simulink model "NONLINEAR_CASE_simulation"  (R2022b)
settings: Solver=ode3  StartTime=0.0  StopTime=15  FixedStep=1e-4  RelTol=1e-6  EnableMultiTasking=on
settings Model: Creator=sf  LastModifiedBy=sf
settings ModelReferenceCC: EnableRefExpFcnMdlSchedulingChecks=on

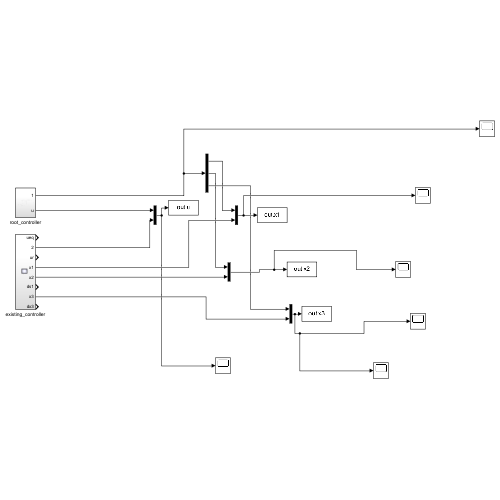
[thumbnail: Simulink's stored preview of the top-level diagram]
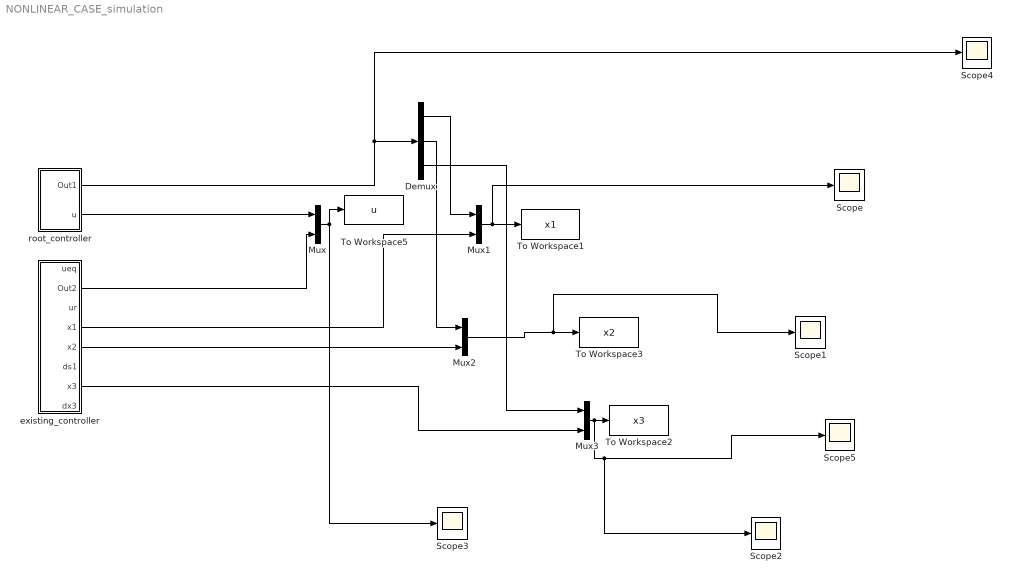
== system NONLINEAR_CASE_simulation ==
  Demux : Demux  Outputs=3
  Mux{,1..3} (4 alike) : Mux  Inputs=2
  Scope{,1..5} (6 alike) : Scope
  To Workspace1 : ToWorkspace  VariableName=x1  SampleTime=-1
  To Workspace2 : ToWorkspace  VariableName=x3  SampleTime=-1
  To Workspace3 : ToWorkspace  VariableName=x2  SampleTime=-1
  To Workspace5 : ToWorkspace  VariableName=u  SampleTime=-1
  existing_controller : Subsystem
  root_controller : Subsystem
  wires:
  root_controller/1(Out1) -> Scope4/1, Demux/1
  root_controller/2(u) -> Mux/1
  existing_controller/2(Out2) -> Mux/2
  existing_controller/4(x1) -> Mux1/2
  Mux/1 -> Scope3/1, To Workspace5/1
  Demux/1 -> Mux1/1
  Demux/2 -> Mux2/1
  existing_controller/5(x2) -> Mux2/2
  Mux2/1 -> Scope1/1, To Workspace3/1
  Demux/3 -> Mux3/1
  existing_controller/7(x3) -> Mux3/2
  Mux3/1 -> Scope2/1, Scope5/1, To Workspace2/1
  Mux1/1 -> Scope/1, To Workspace1/1

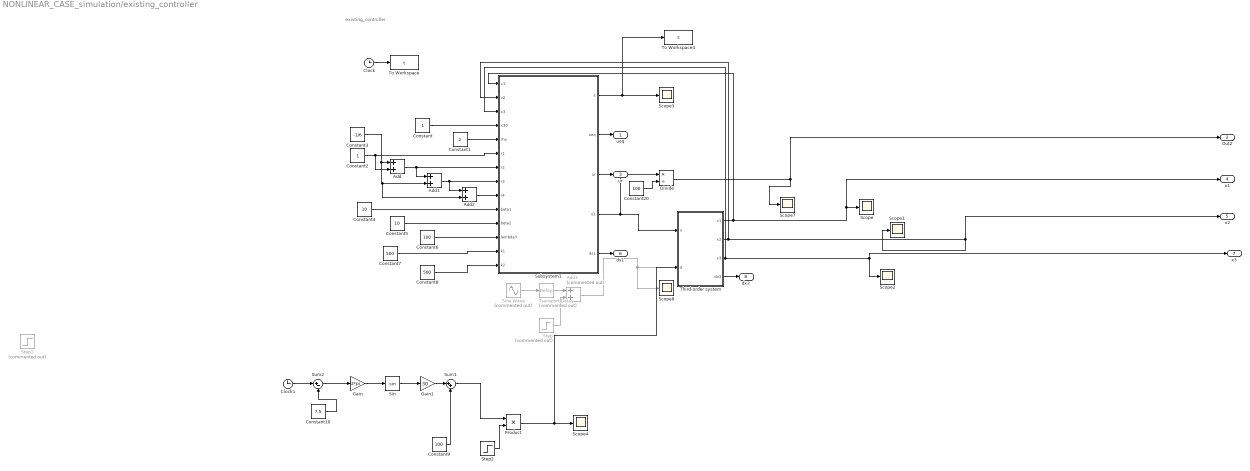
== system NONLINEAR_CASE_simulation/existing_controller ==
  note: existing_controller
  Add : Sum
  Add1 : Sum
  Add2 : Sum
  Add3 : Sum  Commented=on
  Clock : Clock
  Clock1 : Clock
  Constant : Constant
  Constant1 : Constant  Value=2
  Constant10 : Constant  Value=7.5
  Constant2 : Constant
  Constant20 : Constant  Value=100
  Constant3 : Constant  Value=-1/6
  Constant4 : Constant  Value=10
  Constant5 : Constant  Value=10
  Constant6 : Constant  Value=100
  Constant7 : Constant  Value=500
  Constant8 : Constant  Value=500
  Constant9 : Constant  Value=100
  Divide : Product  Inputs=*/
  Gain : Gain  Gain=2*pi
  Gain1 : Gain  Gain=30
  Product : Product
  Scope{,1..4,7..8} (7 alike) : Scope
  Sin : Trigonometry
  Sine Wave : Sin  Commented=on  Amplitude=30  Bias=100  Frequency=2*pi  SampleTime=0
  Step : Step  Commented=on  Time=7.5  After=0  SampleTime=0
  Step1 : Step  Commented=on  Time=7.5  After=0  SampleTime=0
  Step2 : Step  Time=7.5  SampleTime=0
  Subsystem1 : Subsystem
  Sum1 : Sum  Inputs=|++
  Sum2 : Sum  Inputs=|+-
  Third-order system : Subsystem
  To Workspace : ToWorkspace  VariableName=t  SampleTime=-1
  To Workspace4 : ToWorkspace  VariableName=s  SampleTime=-1
  Transport Delay : TransportDelay  Commented=on  DelayTime=7.5
  ueq : Outport
  Out2 : Outport  Port=2
  ur : Outport  Port=3
  x1 : Outport  Port=4
  x2 : Outport  Port=5
  ds1 : Outport  Port=6
  x3 : Outport  Port=7
  dx3 : Outport  Port=8
  wires:
  Third-order system/3(x3) -> x3/1, Scope2/1, Subsystem1/3(x3)
  Subsystem1/3(ur) -> ur/1
  Add/1 -> Add1/1, Subsystem1/7(r2)
  Constant3/1 -> Add2/2, Add1/2, Add/1
  Constant/1 -> Subsystem1/4(x30)
  Constant8/1 -> Subsystem1/14(k2)
  Third-order system/4(dx3) -> dx3/1
  Constant2/1 -> Subsystem1/6(r1), Add/2
  Third-order system/2(x2) -> x2/1, Scope1/1, Subsystem1/2(x2)
  Constant5/1 -> Subsystem1/11(beta2)
  Constant7/1 -> Subsystem1/13(k1)
  Third-order system/1(x1) -> x1/1, Scope/1, Subsystem1/1(x1)
  Subsystem1/4(u1) -> Divide/1, Third-order system/1(u)
  Step/1 -> Add3/2
  Add2/1 -> Subsystem1/9(r4)
  Divide/1 -> Out2/1, Scope7/1
  Constant20/1 -> Divide/2
  Add3/1 -> Scope8/1
  Sine Wave/1 -> Transport Delay/1
  Add1/1 -> Add2/1, Subsystem1/8(r3)
  Constant6/1 -> Subsystem1/12(lambda3)
  Constant1/1 -> Subsystem1/5(rho)
  Subsystem1/1(s) -> To Workspace4/1, Scope3/1
  Transport Delay/1 -> Add3/1
  Clock/1 -> To Workspace/1
  Constant4/1 -> Subsystem1/10(beta1)
  Subsystem1/2(ueq) -> ueq/1
  Subsystem1/5(ds1) -> ds1/1
  Gain/1 -> Sin/1
  Sum1/1 -> Product/1
  Product/1 -> Third-order system/2(d), Scope4/1
  Gain1/1 -> Sum1/1
  Sum2/1 -> Gain/1
  Step2/1 -> Product/2
  Constant9/1 -> Sum1/2
  Sin/1 -> Gain1/1
  Constant10/1 -> Sum2/2
  Clock1/1 -> Sum2/1

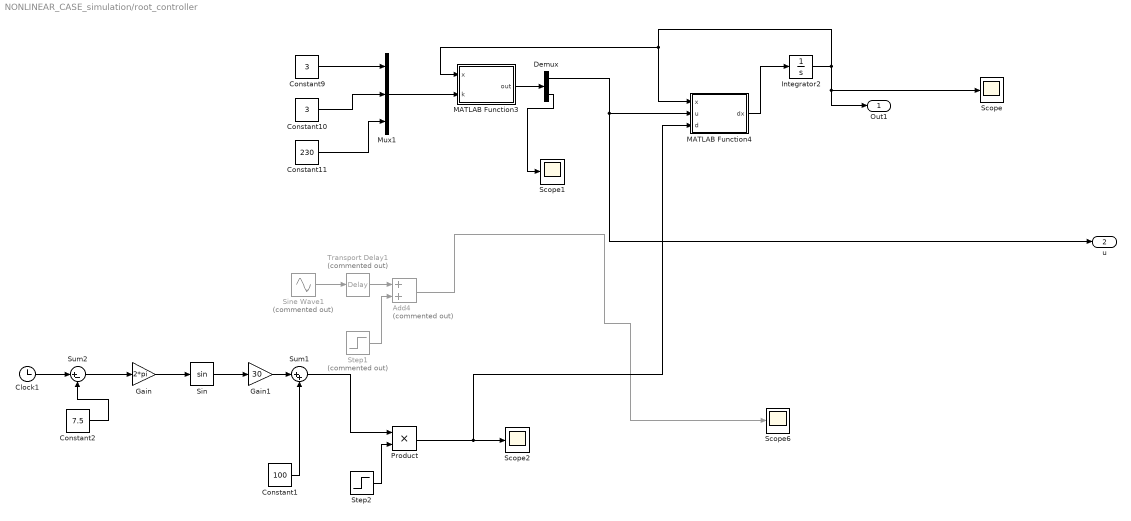
== system NONLINEAR_CASE_simulation/root_controller ==
  Add4 : Sum  Commented=on
  Clock1 : Clock
  Constant1 : Constant  Value=100
  Constant10 : Constant  Value=3
  Constant11 : Constant  Value=230
  Constant2 : Constant  Value=7.5
  Constant9 : Constant  Value=3
  Demux : Demux  Outputs=[1 7]
  Gain : Gain  Gain=2*pi
  Gain1 : Gain  Gain=30
  Integrator2 : Integrator  InitialCondition=[1;1;1]
  MATLAB Function3 : MATLAB Function  TreatAsAtomicUnit=on
  MATLAB Function4 : MATLAB Function  TreatAsAtomicUnit=on
  Mux1 : Mux  Inputs=3
  Product : Product
  Scope{,1..2,6} (4 alike) : Scope
  Sin : Trigonometry
  Sine Wave1 : Sin  Commented=on  Amplitude=30  Bias=100  Frequency=2*pi  SampleTime=0
  Step1 : Step  Commented=on  Time=7.5  After=0  SampleTime=0
  Step2 : Step  Time=7.5  SampleTime=0
  Sum1 : Sum  Inputs=|++
  Sum2 : Sum  Inputs=|+-
  Transport Delay1 : TransportDelay  Commented=on  DelayTime=7.5
  Out1 : Outport
  u : Outport  Port=2
  wires:
  Integrator2/1 -> Scope/1, Out1/1, MATLAB Function3/1(x), MATLAB Function4/1(x)
  Constant11/1 -> Mux1/3
  Constant10/1 -> Mux1/2
  Add4/1 -> Scope6/1
  Constant9/1 -> Mux1/1
  Demux/1 -> u/1, MATLAB Function4/2(u)
  Mux1/1 -> MATLAB Function3/2(k)
  MATLAB Function4/1(dx) -> Integrator2/1
  Sine Wave1/1 -> Transport Delay1/1
  Transport Delay1/1 -> Add4/1
  Step1/1 -> Add4/2
  MATLAB Function3/1(out) -> Demux/1
  Demux/2 -> Scope1/1
  Sin/1 -> Gain1/1
  Constant1/1 -> Sum1/2
  Gain1/1 -> Sum1/1
  Product/1 -> MATLAB Function4/3(d), Scope2/1
  Clock1/1 -> Sum2/1
  Step2/1 -> Product/2
  Constant2/1 -> Sum2/2
  Sum2/1 -> Gain/1
  Sum1/1 -> Product/1
  Gain/1 -> Sin/1

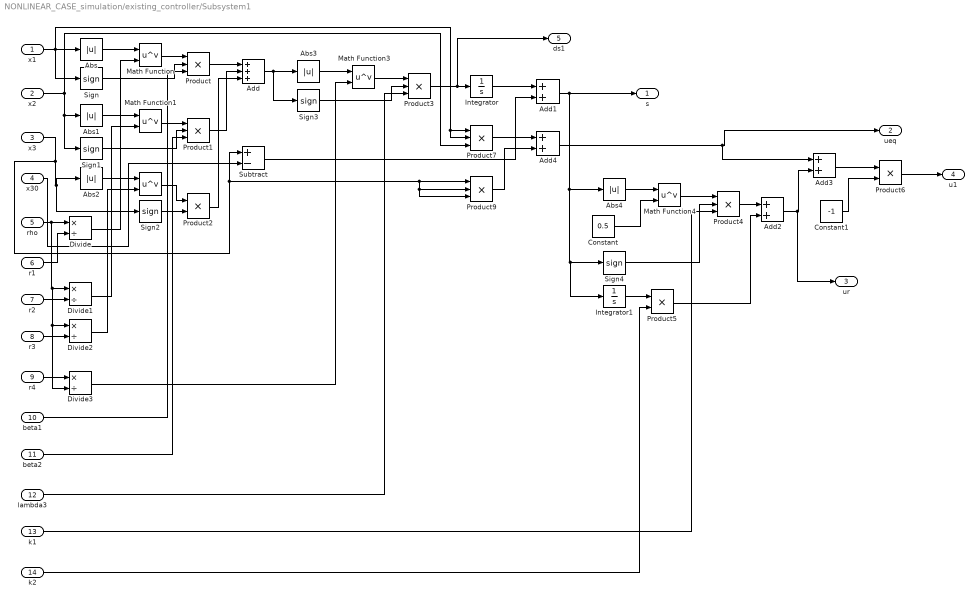
== system NONLINEAR_CASE_simulation/existing_controller/Subsystem1 ==
  x1 : Inport
  x2 : Inport  Port=2
  x3 : Inport  Port=3
  x30 : Inport  Port=4
  rho : Inport  Port=5
  r1 : Inport  Port=6
  r2 : Inport  Port=7
  r3 : Inport  Port=8
  r4 : Inport  Port=9
  beta1 : Inport  Port=10
  beta2 : Inport  Port=11
  lambda3 : Inport  Port=12
  k1 : Inport  Port=13
  k2 : Inport  Port=14
  " " : Math  Operator=pow  SignedPower=on
  Abs{,1..4} (5 alike) : Abs  SaturateOnIntegerOverflow=off
  Add : Sum  Inputs=+++
  Add{1..4} (4 alike) : Sum
  Constant : Constant  Value=0.5
  Constant1 : Constant  Value=-1
  Divide{,1..3} (4 alike) : Product  Inputs=*/
  Integrator : Integrator
  Integrator1 : Integrator
  Math Function{,1,3..4} (4 alike) : Math  Operator=pow  SignedPower=on
  Product{,1,3..4,7,9} (6 alike) : Product  Inputs=3
  Product2 : Product
  Product5 : Product
  Product6 : Product
  Sign{,1..4} (5 alike) : Signum
  Subtract : Sum  Inputs=+-
  s : Outport
  ueq : Outport  Port=2
  ur : Outport  Port=3
  u1 : Outport  Port=4
  ds1 : Outport  Port=5
  wires:
  k2/1 -> Product5/2
  Add3/1 -> Product6/1
  Constant/1 -> Math Function4/2
  x1/1 -> Sign/1, Product7/2, Product7/1, Abs/1
  lambda3/1 -> Product3/3
  Math Function4/1 -> Product4/1
  Constant1/1 -> Product6/2
  Abs4/1 -> Math Function4/1
  Abs/1 -> Math Function/1
  Math Function/1 -> Product/1
  Sign1/1 -> Product1/2
  Divide3/1 -> Math Function3/2
  " "/1 -> Product2/1
  rho/1 -> Divide3/2, Divide2/1, Divide1/1, Divide/1
  Abs3/1 -> Math Function3/1
  Abs2/1 -> " "/1
  Sign2/1 -> Product2/2
  Product1/1 -> Add/2
  r1/1 -> Divide/2
  r3/1 -> Divide2/2
  x2/1 -> Sign1/1, Abs1/1, Product7/3
  beta2/1 -> Product1/3
  x3/1 -> Product9/3, Product9/2, Product9/1, Subtract/1, Sign2/1, Abs2/1
  Abs1/1 -> Math Function1/1
  Product/1 -> Add/1
  Divide2/1 -> " "/2
  Add/1 -> Sign3/1, Abs3/1
  Product2/1 -> Add/3
  Sign4/1 -> Product4/2
  Product5/1 -> Add2/2
  Sign3/1 -> Product3/2
  Product4/1 -> Add2/1
  Integrator/1 -> Add1/1
  r4/1 -> Divide3/1
  Integrator1/1 -> Product5/1
  Math Function3/1 -> Product3/1
  Product3/1 -> ds1/1, Integrator/1
  Subtract/1 -> Add1/2
  Add1/1 -> s/1, Integrator1/1, Sign4/1, Abs4/1
  x30/1 -> Subtract/2
  Add2/1 -> ur/1, Add3/2
  Divide/1 -> Math Function/2
  Divide1/1 -> Math Function1/2
  k1/1 -> Product4/3
  Math Function1/1 -> Product1/1
  r2/1 -> Divide1/2
  beta1/1 -> Product/3
  Sign/1 -> Product/2
  Product7/1 -> Add4/1
  Product9/1 -> Add4/2
  Add4/1 -> Add3/1, ueq/1
  Product6/1 -> u1/1

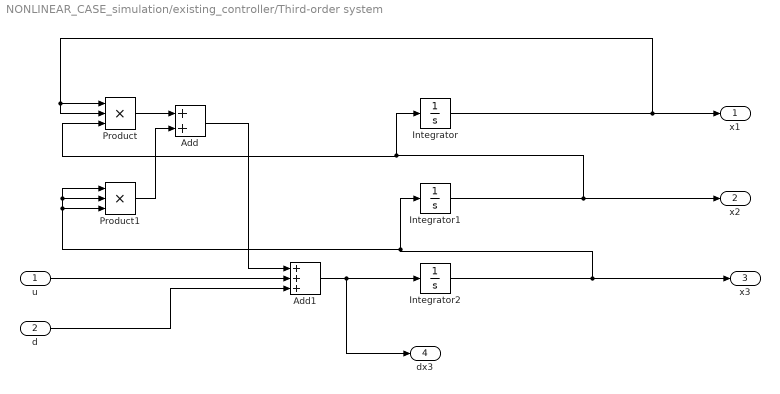
== system NONLINEAR_CASE_simulation/existing_controller/Third-order system ==
  u : Inport
  d : Inport  Port=2
  Add : Sum
  Add1 : Sum  Inputs=+++
  Integrator : Integrator  InitialCondition=1
  Integrator1 : Integrator  InitialCondition=1
  Integrator2 : Integrator  InitialCondition=1
  Product : Product  Inputs=3
  Product1 : Product  Inputs=3
  x1 : Outport
  x2 : Outport  Port=2
  x3 : Outport  Port=3
  dx3 : Outport  Port=4
  wires:
  Integrator/1 -> Product/2, Product/1, x1/1
  Integrator2/1 -> x3/1, Product1/3, Product1/1, Product1/2, Integrator1/1
  Integrator1/1 -> x2/1, Product/3, Integrator/1
  Product/1 -> Add/1
  Product1/1 -> Add/2
  Add1/1 -> dx3/1, Integrator2/1
  Add/1 -> Add1/1
  u/1 -> Add1/2
  d/1 -> Add1/3

== matlab function NONLINEAR_CASE_simulation/root_controller/MATLAB Function4 ==
  data: x input; u input; dx output; d input
function dx = fcn(x,u,d)
x1 = x(1);
x2 = x(2);
x3 = x(3);
x1dot = x2;
x2dot = x3;
x3dot =100*u+x1^2*x2+x3^3+d;
dx = [x1dot;x2dot;x3dot];

== matlab function NONLINEAR_CASE_simulation/root_controller/MATLAB Function3 ==
  data: x input; out output; k input
function out = fcn(x,k)
x1 = x(1);
x2 = x(2);
x3 = x(3);
x1dot = x2;
x2dot = x3;
k1 = k(1);
k2 = k(2);
k3 = k(3);
% a,b,c,d>0, x^r>0
% a>b concave function
% a<b convex function
% Fcr = (c*x^r+a)/(d*x^r+b)*x;

% x1
a1 =0.3;
b1 = 0.1;
c1 =0.5 ;
d1 =1;
r1 = 1;
f1 = fcrt(x1,a1,b1,c1,d1,r1);
x2d = -k1*f1;
f1dx = fcrtdot(x1,a1,b1,c1,d1,r1);
x2ddot = -k1*f1dx*x1dot;
f1ddx= fcrtddot(x1,a1,b1,c1,d1,r1);
x2dddot =-k1*f1ddx*x1dot*x1dot-k1*f1dx*x2dot;
% x2
a2 = 0.35;
b2 = 0.0008;
c2 =0.1;
d2 = 2.9;
r2 = 1;
e2 = x2-x2d;
f2 = fcrt(e2,a2,b2,c2,d2,r2);
x3d = -k2*f2+x2ddot-x1;
f2dx = fcrtdot(e2,a2,b2,c2,d2,r2);
%f2dx = min(max(f2dx,-10),10);
%f22dx = fcrtdot(e2,b2,a2,c2,d2,r2);
x3ddot = -k2*(f2dx)*(x2dot-x2ddot)+x2dddot-x1dot;
% x3
a3 = 9;
b3 = 0.00001;
c3 =0.4;
d3 =0.55;
r3 = 3;
e3 = x3-x3d;
f3 = fcrt2(e3,a3,b3,c3,d3,r3);
u = (-k3*(f3)-(abs(e3)+0.08)/(abs(e3)+0.0001)*e3+x3ddot-e2-x1^2*x2-x3^3)/100;
out=[u;e2;e3;x2ddot;x2dddot;x3ddot;f2dx;f1dx];
end

function y = fcrt(x, a, b, c, d, r)
y = (c*x^r+a)/(d*x^r+b)*x;
%y= (c*abs(x)^r)/(d*abs(x)^r+b)*nthroot(x,a);
end

function y = fcrt2(x, a, b, c, d, r)
%y = (c*x^r+a)/(d*x^r+b)*x;
y= (c*abs(x)^r)/(d*abs(x)^r+b)*nthroot(x,a);
end

function ydot = fcrtdot(x, a, b, c, d, r)
ydot =(a + c*x^r)/(b + d*x^r+eps) + (c*r*x*x^(r - 1))/(b + d*x^r+eps) - (d*r*x*x^(r - 1)*(a + c*x^r))/(b + d*x^r+eps)^2;
%ydot=(c*r*abs(x)^(r - 1)*sign(x)*nthroot(x, a))/(b + d*abs(x)^r) + (c*abs(x)^r*nthroot(x, a))/(a*x*(b + d*abs(x)^r)) - (c*d*r*abs(x)^(r - 1)*abs(x)^r*sign(x)*nthroot(x, a))/(b + d*abs(x)^r)^2;
end

function ydot = fcrtdot2(x, a, b, c, d, r)
%ydot =(a + c*x^r)/(b + d*x^r+eps) + (c*r*x*x^(r - 1))/(b + d*x^r+eps) - (d*r*x*x^(r - 1)*(a + c*x^r))/(b + d*x^r+eps)^2;
ydot=(c*r*abs(x)^(r - 1)*sign(x)*nthroot(x, a))/(b + d*abs(x)^r) + (c*abs(x)^r*nthroot(x, a))/(a*x*(b + d*abs(x)^r)) - (c*d*r*abs(x)^(r - 1)*abs(x)^r*sign(x)*nthroot(x, a))/(b + d*abs(x)^r)^2;
end
 
function yddot = fcrtddot(x, a, b, c, d, r)
yddot =(2*c*r*x^(r - 1))/(b + d*x^r+eps) - (2*d*r*x^(r - 1)*(a + c*x^r))/(b + d*x^r+eps)^2 + (c*r*x*x^(r - 2)*(r - 1))/(b + d*x^r+eps) + (2*d^2*r^2*x*x^(2*r - 2)*(a + c*x^r))/(b + d*x^r+eps)^3 - (2*c*d*r^2*x*x^(2*r - 2))/(b + d*x^r+eps)^2 - (d*r*x*x^(r - 2)*(a + c*x^r)*(r - 1))/(b + d*x^r+eps)^2;
%yddot=(c*abs(x)^r*nthroot(x, a))/(a^2*x^2*(b + d*abs(x)^r)) - (c*abs(x)^r*nthroot(x, a))/(a*x^2*(b + d*abs(x)^r))  + (c*r*abs(x)^(r - 2)*sign(x)^2*nthroot(x, a)*(r - 1))/(b + d*abs(x)^r) - (2*c*d*r^2*abs(x)^(2*r - 2)*sign(x)^2*nthroot(x, a))/(b + d*abs(x)^r)^2  + (2*c*d^2*r^2*abs(x)^(2*r - 2)*abs(x)^r*sign(x)^2*nthroot(x, a))/(b + d*abs(x)^r)^3 + (2*c*r*abs(x)^(r - 1)*sign(x)*nthroot(x, a))/(a*x*(b + d*abs(x)^r)) - (c*d*r*abs(x)^(r - 2)*abs(x)^r*sign(x)^2*nthroot(x, a)*(r - 1))/(b + d*abs(x)^r)^2 - (2*c*d*r*abs(x)^(r - 1)*abs(x)^r*sign(x)*nthroot(x, a))/(a*x*(b + d*abs(x)^r)^2);

end

function yddot = fcrtddot2(x, a, b, c, d, r)
%yddot =(2*c*r*x^(r - 1))/(b + d*x^r+eps) - (2*d*r*x^(r - 1)*(a + c*x^r))/(b + d*x^r+eps)^2 + (c*r*x*x^(r - 2)*(r - 1))/(b + d*x^r+eps) + (2*d^2*r^2*x*x^(2*r - 2)*(a + c*x^r))/(b + d*x^r+eps)^3 - (2*c*d*r^2*x*x^(2*r - 2))/(b + d*x^r+eps)^2 - (d*r*x*x^(r - 2)*(a + c*x^r)*(r - 1))/(b + d*x^r+eps)^2;
yddot=(c*abs(x)^r*nthroot(x, a))/(a^2*x^2*(b + d*abs(x)^r)) - (c*abs(x)^r*nthroot(x, a))/(a*x^2*(b + d*abs(x)^r))  + (c*r*abs(x)^(r - 2)*sign(x)^2*nthroot(x, a)*(r - 1))/(b + d*abs(x)^r) - (2*c*d*r^2*abs(x)^(2*r - 2)*sign(x)^2*nthroot(x, a))/(b + d*abs(x)^r)^2  + (2*c*d^2*r^2*abs(x)^(2*r - 2)*abs(x)^r*sign(x)^2*nthroot(x, a))/(b + d*abs(x)^r)^3 + (2*c*r*abs(x)^(r - 1)*sign(x)*nthroot(x, a))/(a*x*(b + d*abs(x)^r)) - (c*d*r*abs(x)^(r - 2)*abs(x)^r*sign(x)^2*nthroot(x, a)*(r - 1))/(b + d*abs(x)^r)^2 - (2*c*d*r*abs(x)^(r - 1)*abs(x)^r*sign(x)*nthroot(x, a))/(a*x*(b + d*abs(x)^r)^2);

end
